simulink model "Jordan"  (R2018b)
settings: Solver=VariableStepAuto  StartTime=0.0  StopTime=10.0  RelTol=1e-3
settings Model: Creator=kekos  LastModifiedBy=kekos

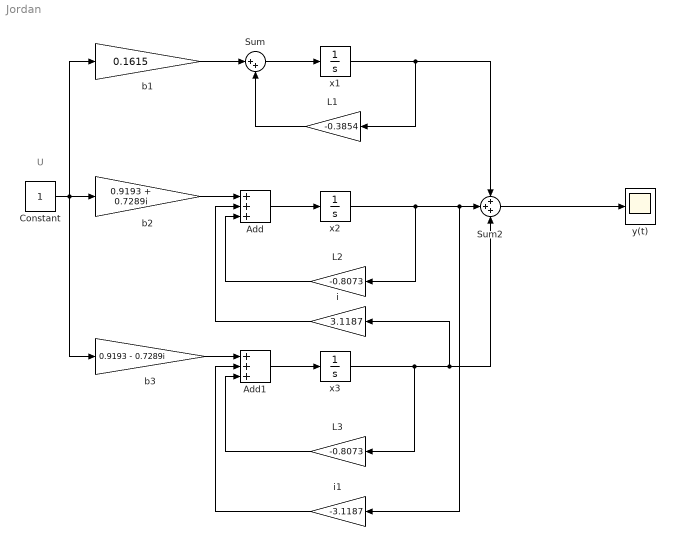
== system Jordan ==
  note: U
  Add : Sum  Inputs=3
  Add1 : Sum  Inputs=3
  Constant : Constant
  L1 : Gain  Gain=-0.3854
  L2 : Gain  Gain=-0.8073
  L3 : Gain  Gain=-0.8073
  Sum : Sum  Inputs=|++
  Sum2 : Sum  Inputs=+++
  b1 : Gain  Gain=0.1615
  b2 : Gain  Gain=0.9193 + 0.7289i
  b3 : Gain  Gain=0.9193 - 0.7289i
  i : Gain  Gain=3.1187
  i1 : Gain  Gain=-3.1187
  x1 : Integrator  InitialCondition=1
  x2 : Integrator  InitialCondition=1
  x3 : Integrator  InitialCondition=1
  y(t) : Scope
  wires:
  Constant/1 -> b1/1, b3/1, b2/1
  b1/1 -> Sum/1
  Sum/1 -> x1/1
  x1/1 -> Sum2/1, L1/1
  L1/1 -> Sum/2
  Sum2/1 -> y(t)/1
  x2/1 -> L2/1, i1/1, Sum2/2
  x3/1 -> L3/1, i/1, Sum2/3
  b2/1 -> Add/1
  Add/1 -> x2/1
  L2/1 -> Add/3
  i/1 -> Add/2
  b3/1 -> Add1/1
  Add1/1 -> x3/1
  L3/1 -> Add1/3
  i1/1 -> Add1/2
